simulink model "tema_2017"  (R2017a)
settings: Solver=VariableStepAuto  StartTime=0.0  StopTime=10.0  RelTol=1e-3
values from neighbouring files (symbols this model uses):
  A1 = 0.06    [load_workspace_a.m]    (also in load_workspace_b.m; load_workspace_c.m; load_workspace_d.m; load_workspace_e.m)
  a1 = 1.31 / 10^4    (= 0.000131)    [load_workspace_a.m]    (also in load_workspace_b.m; load_workspace_c.m; load_workspace_d.m; load_workspace_e.m)
  A2 = 0.06    [load_workspace_a.m]    (also in load_workspace_b.m; load_workspace_c.m; load_workspace_d.m; load_workspace_e.m)
  a2 = 1.51 / 10^4    (= 0.000151)    [load_workspace_a.m]    (also in load_workspace_b.m; load_workspace_c.m; load_workspace_d.m; load_workspace_e.m)
  A3 = 0.06    [load_workspace_a.m]    (also in load_workspace_b.m; load_workspace_c.m; load_workspace_d.m; load_workspace_e.m)
  a3 = 9.27 / 10^5    (= 9.27e-05)    [load_workspace_a.m]    (also in load_workspace_b.m; load_workspace_c.m; load_workspace_d.m; load_workspace_e.m)
  A4 = 0.06    [load_workspace_a.m]    (also in load_workspace_b.m; load_workspace_c.m; load_workspace_d.m; load_workspace_e.m)
  a4 = 8.82 / 10^5    (= 8.82e-05)    [load_workspace_a.m]    (also in load_workspace_b.m; load_workspace_c.m; load_workspace_d.m; load_workspace_e.m)
  ac = 4.307 / 10^6    (= 4.307e-06)    [load_workspace_a.m]    (also in load_workspace_b.m; load_workspace_c.m; load_workspace_d.m; load_workspace_e.m)
  amp_u1 = 1    [load_workspace_a.m]    (also in load_workspace_b.m; load_workspace_c.m; load_workspace_d.m = 2; load_workspace_e.m = 2)
  amp_u2 = 1    [load_workspace_a.m]    (also in load_workspace_b.m; load_workspace_c.m; load_workspace_d.m = 4; load_workspace_e.m = 4)
  AT = 0.1273    [load_workspace_a.m]    (also in load_workspace_b.m; load_workspace_c.m; load_workspace_d.m; load_workspace_e.m)
  cih = 1    [load_workspace_a.m]    (also in load_workspace_c.m; load_workspace_d.m; load_workspace_e.m; load_workspace_f.m)
  cih1 = 0    [load_workspace_a.m]    (also in load_workspace_c.m; load_workspace_d.m; load_workspace_e.m; load_workspace_f.m)
  cih2 = 0    [load_workspace_a.m]    (also in load_workspace_c.m; load_workspace_d.m; load_workspace_e.m; load_workspace_f.m)
  cih3 = 0    [load_workspace_a.m]    (also in load_workspace_c.m; load_workspace_d.m; load_workspace_e.m; load_workspace_f.m)
  cih4 = 0    [load_workspace_a.m]    (also in load_workspace_c.m; load_workspace_d.m; load_workspace_e.m; load_workspace_f.m)
  g = 9.8    [load_workspace_a.m]    (also in load_workspace_b.m; load_workspace_c.m; load_workspace_d.m; load_workspace_e.m)
  kp = 0.5 / 10^4    (= 5e-05)    [load_workspace_a.m]    (also in load_workspace_b.m; load_workspace_c.m; load_workspace_d.m; load_workspace_e.m)
  l1 = 2/4    (= 0.5)    [load_workspace_a.m]    (also in load_workspace_b.m; load_workspace_c.m; load_workspace_d.m; load_workspace_e.m)
  l2 = 3/4    (= 0.75)    [load_workspace_a.m]    (also in load_workspace_b.m; load_workspace_c.m; load_workspace_d.m; load_workspace_e.m)
  q = 1000    [load_workspace_a.m]    (also in load_workspace_b.m; load_workspace_c.m; load_workspace_d.m; load_workspace_e.m)
  step1 = 2    [load_workspace_a.m]    (also in load_workspace_b.m; load_workspace_c.m; load_workspace_d.m; load_workspace_e.m)
  step2 = 1    [load_workspace_a.m]    (also in load_workspace_b.m; load_workspace_c.m; load_workspace_d.m; load_workspace_e.m)
settings Model: Creator=pangi  LastModifiedBy=ialex

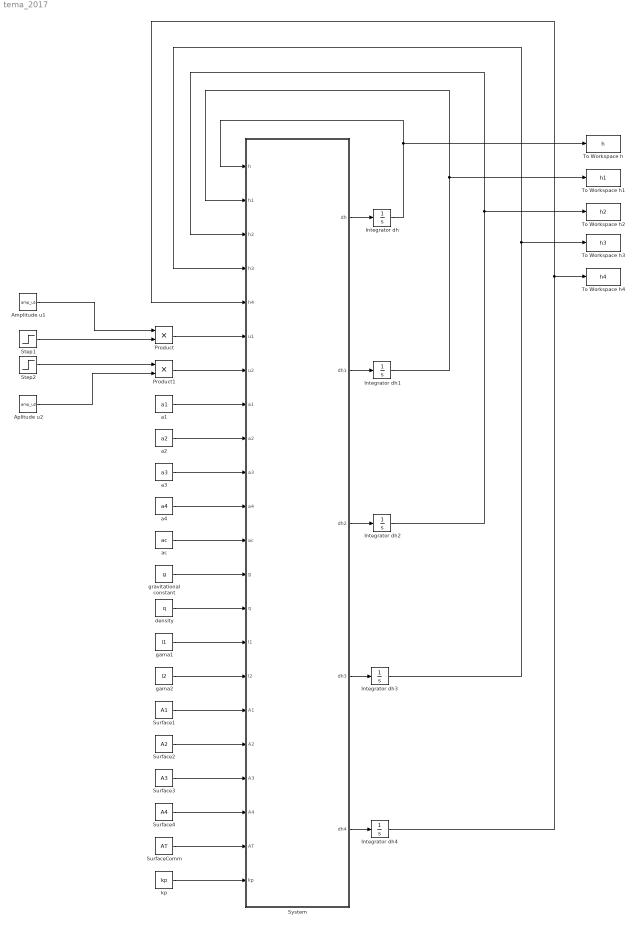
== system tema_2017 ==
  " gama1" : Constant  Value=l1  VectorParams1D=off
  Amplitude u1 : Constant  Value=amp_u1
  Aplitude u2 : Constant  Value=amp_u2
  Integrator dh : Integrator  InitialCondition=cih
  Integrator dh1 : Integrator  InitialCondition=cih1
  Integrator dh2 : Integrator  InitialCondition=cih2
  Integrator dh3 : Integrator  InitialCondition=cih3
  Integrator dh4 : Integrator  InitialCondition=cih4
  Product : Product
  Product1 : Product
  Step1 : Step  After=step1  SampleTime=0
  Step2 : Step  After=step2  SampleTime=0
  Surface1 : Constant  Value=A1  VectorParams1D=off
  Surface2 : Constant  Value=A2  VectorParams1D=off
  Surface3 : Constant  Value=A3  VectorParams1D=off
  Surface4 : Constant  Value=A4  VectorParams1D=off
  SurfaceComm : Constant  Value=AT  VectorParams1D=off
  System : MATLAB Function  TreatAsAtomicUnit=on
  To Workspace h : ToWorkspace  VariableName=h  SaveFormat=Timeseries  SampleTime=-1
  To Workspace h1 : ToWorkspace  VariableName=h1  SaveFormat=Timeseries  SampleTime=-1
  To Workspace h2 : ToWorkspace  VariableName=h2  SaveFormat=Timeseries  SampleTime=-1
  To Workspace h3 : ToWorkspace  VariableName=h3  SaveFormat=Timeseries  SampleTime=-1
  To Workspace h4 : ToWorkspace  VariableName=h4  SaveFormat=Timeseries  SampleTime=-1
  a1 : Constant  Value=a1  VectorParams1D=off
  a2 : Constant  Value=a2  VectorParams1D=off
  a3 : Constant  Value=a3  VectorParams1D=off
  a4 : Constant  Value=a4  VectorParams1D=off
  ac : Constant  Value=ac  VectorParams1D=off
  density : Constant  Value=q  VectorParams1D=off
  gama2 : Constant  Value=l2  VectorParams1D=off
  gravitational constant : Constant  Value=g  VectorParams1D=off
  kp : Constant  Value=kp  VectorParams1D=off
  wires:
  a1/1 -> System/8(a1)
  a2/1 -> System/9(a2)
  a3/1 -> System/10(a3)
  a4/1 -> System/11(a4)
  ac/1 -> System/12(ac)
  gravitational constant/1 -> System/13(g)
  density/1 -> System/14(q)
  " gama1"/1 -> System/15(l1)
  gama2/1 -> System/16(l2)
  Surface1/1 -> System/17(A1)
  Surface2/1 -> System/18(A2)
  Surface3/1 -> System/19(A3)
  Surface4/1 -> System/20(A4)
  SurfaceComm/1 -> System/21(AT)
  kp/1 -> System/22(kp)
  System/1(dh) -> Integrator dh/1
  System/2(dh1) -> Integrator dh1/1
  System/4(dh3) -> Integrator dh3/1
  System/5(dh4) -> Integrator dh4/1
  System/3(dh2) -> Integrator dh2/1
  Integrator dh4/1 -> System/5(h4), To Workspace h4/1
  Integrator dh3/1 -> To Workspace h3/1, System/4(h3)
  Integrator dh2/1 -> To Workspace h2/1, System/3(h2)
  Integrator dh1/1 -> To Workspace h1/1, System/2(h1)
  Integrator dh/1 -> To Workspace h/1, System/1(h)
  Step1/1 -> Product/2
  Step2/1 -> Product1/1
  Aplitude u2/1 -> Product1/2
  Amplitude u1/1 -> Product/1
  Product/1 -> System/6(u1)
  Product1/1 -> System/7(u2)

== matlab function tema_2017/System ==
  data: dh output; h input; h1 input; h2 input; h3 input; h4 input; u1 input; dh1 output; dh2 output; dh3 output; dh4 output; u2 input; a1 input; a2 input; a3 input; a4 input; ac input; g input; q input; l1 input; l2 input; A1 input; A2 input; A3 input; A4 input; AT input; kp input
function [dh, dh1, dh2, dh3, dh4] = fcn(h, h1, h2, h3, h4, u1, u2, a1, a2, a3, a4, ac, g, q, l1, l2, A1, A2, A3, A4, AT, kp)
    dh1 = 1/A1*(-a1*sqrt(2*g*h1) - ac*sign(q*g*h1 - q*g*h2)*sqrt(2*g*abs(h1 - h2)) + a3*sqrt(2*g*h3) + l1*kp*u1);
    dh2 = 1/A2*(-a2*sqrt(2*g*h2) - ac*sign(q*g*h1 - q*g*h2)*sqrt(2*g*abs(h1 - h2)) + a4*sqrt(2*g*h4) + l2*kp*u2);
    dh3 = 1/A3*(-a3*sqrt(2*g*h3) + (1 - l2)*kp*u2);
    dh4 = 1/A4*(-a4*sqrt(2*g*h4) + (1 - l1)*kp*u1);
    dh = 1/AT*(a1*sqrt(2*g*h1) + a2*sqrt(2*g*h2) - kp*u1 - kp*u2);
end
